simulink model "DC_Servo_S"  (R2013a)
settings: Solver=ode45  StartTime=0.0  StopTime=10.0  RelTol=1e-3
undefined symbols (not defined in the file): b, j, kb, kt, L, R
settings Model: Creator=Ahmed  LastModifiedBy=Ahmed

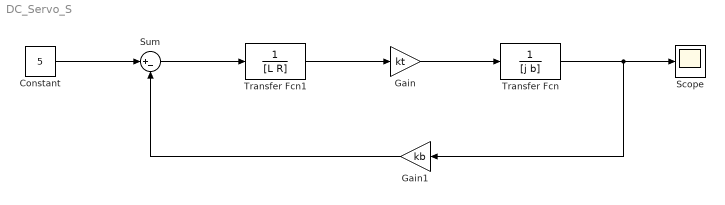
== system DC_Servo_S ==
  Constant : Constant  Value=5
  Gain : Gain  Gain=kt
  Gain1 : Gain  Gain=kb
  Scope : Scope
  Sum : Sum  Inputs=|+-
  Transfer Fcn : TransferFcn  Denominator=[j b]
  Transfer Fcn1 : TransferFcn  Denominator=[L R]
  wires:
  Constant/1 -> Sum/1
  Sum/1 -> Transfer Fcn1/1
  Transfer Fcn1/1 -> Gain/1
  Gain/1 -> Transfer Fcn/1
  Transfer Fcn/1 -> Gain1/1, Scope/1
  Gain1/1 -> Sum/2
